simulink model "posdcmotor"  (R2017b)
settings: Solver=FixedStepDiscrete  StartTime=0.0  StopTime=inf  RelTol=1e-3  EnableMultiTasking=on
undefined symbols (not defined in the file): DiscIntNeverNeededParam
libraries: arduinolib x3, simulink x1, instrumentlib x1
settings Model: ExtModeTrigDuration=2  Creator=Caue  LastModifiedBy=gmore
settings OptimizationCC: PassReuseOutputArgsThreshold=0  MaxStackSize=64
settings DebuggingCC: ParameterTunabilityLossMsg=error
settings HardwareCC: ProdBitPerInt=16  ProdBitPerPointer=16  ProdBitPerSizeT=16  ProdBitPerPtrDiffT=16  ProdLargestAtomicFloat=None  ProdWordSize=8  ProdHWDeviceType=Atmel->AVR  UseEmbeddedCoderFeatures=off  UseSimulinkCoderFeatures=off
settings SFSimCC: MATLABDynamicMemAlloc=off
settings RTWCC: SystemTargetFile=ert.tlc  HardwareBoard=Arduino Uno  TLCOptions=-aInlineSetEventsForThisBaseRateFcn=TLC_FALSE -aSuppressMultiTaskScheduler=TLC_FALSE -aRateBasedStepFcn=1  TemplateMakefile=ert_default_tmf  GenerateReport=on  Toolchain=Arduino AVR  BuildConfiguration=Faster Runs  LaunchReport=on
settings CodeAppCC: ForceParamTrailComments=on  OperatorAnnotations=on  StateflowObjectComments=on  MATLABSourceComments=on
settings ERTTargetCC: ERTCustomFileBanners=off  SupportContinuousTime=on  SupportNonInlinedSFcns=on  RemoveResetFunc=off  SupportVariableSizeSignals=on  ModelStepFunctionPrototypeControlCompliant=off

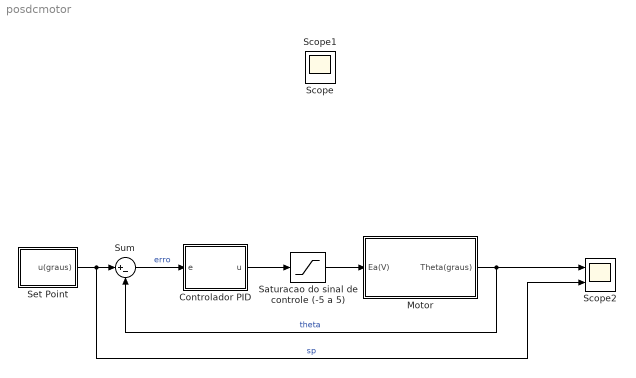
== system posdcmotor ==
  Controlador PID : Subsystem  mask{Kp=1.0, Kd=0.0, Ki=0.0}
  Motor : Subsystem
  Saturacao do sinal de controle (-5 a 5) : Saturate  UpperLimit=5  LowerLimit=-5
  Scope2 : Scope  NumInputPorts=2
  Set Point : Subsystem
  Sum : Sum  Inputs=|+-
  Scope : Scope
  Scope1 : Scope
  wires:
  Motor/1(Theta(graus)) -> Scope2/1, Sum/2  "theta"
  Set Point/1(u(graus)) -> Scope2/2, Sum/1  "sp"
  Saturacao do sinal de controle (-5 a 5)/1 -> Motor/1(Ea(V))
  Sum/1 -> Controlador PID/1(e)  "erro"
  Controlador PID/1(u) -> Saturacao do sinal de controle (-5 a 5)/1

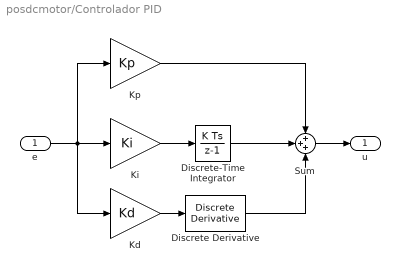
== system posdcmotor/Controlador PID ==
  e : Inport
  Discrete Derivative : simulink/Discrete/Discrete Derivative  gainval=1.0  ICPrevScaledInput=0.0  OutMin=[]  OutMax=[]  OutDataType=fixdt(1, 16)  OutScaling=2^-10  DoSatur=off
  Discrete-Time Integrator : DiscreteIntegrator  InitialConditionSetting=State (most efficient)  SampleTime=-1  ICPrevOutput=DiscIntNeverNeededParam  ICPrevScaledInput=DiscIntNeverNeededParam
  Kd : Gain  Gain=Kd
  Ki : Gain  Gain=Ki
  Kp : Gain  Gain=Kp
  Sum : Sum  Inputs=+++
  u : Outport
  wires:
  e/1 -> Kp/1, Kd/1, Ki/1
  Ki/1 -> Discrete-Time Integrator/1
  Kd/1 -> Discrete Derivative/1
  Sum/1 -> u/1
  Discrete-Time Integrator/1 -> Sum/2
  Kp/1 -> Sum/1
  Discrete Derivative/1 -> Sum/3

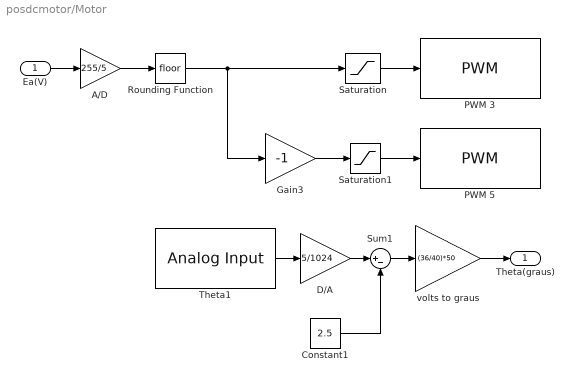
== system posdcmotor/Motor ==
  Ea(V) : Inport
  A/D : Gain  Gain=255/5
  Constant1 : Constant  Value=2.5
  D/A : Gain  Gain=5/1024
  Gain3 : Gain  Gain=-1
  PWM 3 : arduinolib/PWM  pinNumber=3  blockPlatform=arduino
  PWM 5 : arduinolib/PWM  pinNumber=5  blockPlatform=arduino
  Rounding Function : Rounding
  Saturation : Saturate  UpperLimit=255  LowerLimit=0
  Saturation1 : Saturate  UpperLimit=255  LowerLimit=0
  Sum1 : Sum  Inputs=|+-
  Theta1 : arduinolib/Analog Input  pinNumber=1  sampleTime=0.02  blockPlatform=arduino
  volts to graus : Gain  Gain=(36/40)*50
  Theta(graus) : Outport
  wires:
  A/D/1 -> Rounding Function/1
  Gain3/1 -> Saturation1/1
  Saturation/1 -> PWM 3/1
  Rounding Function/1 -> Gain3/1, Saturation/1
  D/A/1 -> Sum1/1
  Sum1/1 -> volts to graus/1
  volts to graus/1 -> Theta(graus)/1
  Constant1/1 -> Sum1/2
  Saturation1/1 -> PWM 5/1
  Theta1/1 -> D/A/1
  Ea(V)/1 -> A/D/1

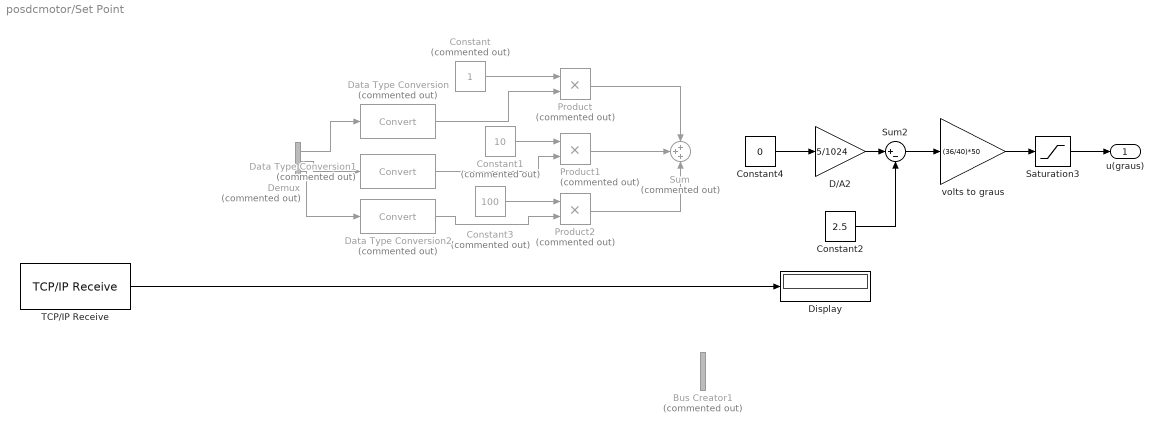
== system posdcmotor/Set Point ==
  Bus Creator1 : BusCreator  Commented=on  Inputs=3
  Constant : Constant  Commented=on  OutDataTypeStr=uint8
  Constant1 : Constant  Commented=on  Value=10  OutDataTypeStr=uint8
  Constant2 : Constant  Value=2.5
  Constant3 : Constant  Commented=on  Value=100  OutDataTypeStr=uint8
  Constant4 : Constant  Value=0
  D/A2 : Gain  Gain=5/1024
  Data Type Conversion : DataTypeConversion  Commented=on
  Data Type Conversion1 : DataTypeConversion  Commented=on
  Data Type Conversion2 : DataTypeConversion  Commented=on
  Demux : Demux  Commented=on  Outputs=3
  Display : Display
  Product : Product  Commented=on
  Product1 : Product  Commented=on
  Product2 : Product  Commented=on
  Saturation3 : Saturate  UpperLimit=100  LowerLimit=-100
  Sum : Sum  Commented=on  Inputs=+++
  Sum2 : Sum  Inputs=|+-
  TCP/IP Receive : instrumentlib/TCP//IP Receive  Host=10.92.106.119  Port=4321  DataSize="[1  1]"  EnableBlockingMode=on  Timeout=10  SampleTime=0.02  DataType=single  ByteOrder=BigEndian
      settings: SourceProductName=Instrument Control Toolbox
  volts to graus : Gain  Gain=(36/40)*50
  u(graus) : Outport
  wires:
  Saturation3/1 -> u(graus)/1
  Constant2/1 -> Sum2/2
  D/A2/1 -> Sum2/1
  volts to graus/1 -> Saturation3/1
  Sum2/1 -> volts to graus/1
  Demux/2 -> Data Type Conversion1/1
  Demux/1 -> Data Type Conversion/1
  Demux/3 -> Data Type Conversion2/1
  Constant/1 -> Product/1
  Data Type Conversion/1 -> Product/2
  Data Type Conversion1/1 -> Product1/2
  Constant1/1 -> Product1/1
  Data Type Conversion2/1 -> Product2/2
  Constant3/1 -> Product2/1
  Product/1 -> Sum/1
  Product2/1 -> Sum/3
  Product1/1 -> Sum/2
  Constant4/1 -> D/A2/1
  TCP/IP Receive/1 -> Display/1
